simulink model "Architecture"  (R2016b)
settings: Solver=VariableStepAuto  StartTime=0.0  StopTime=10.0  RelTol=1e-3
settings Model: Creator=Taeke  LastModifiedBy=Taeke

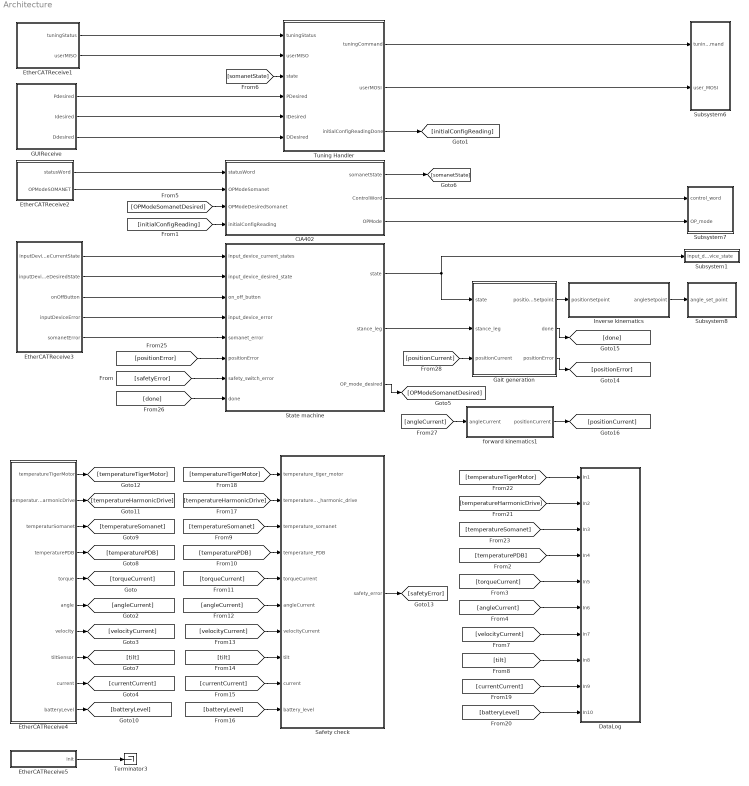
== system Architecture ==
  CiA402 : MATLAB Function  TreatAsAtomicUnit=on
  DataLog : Subsystem
  EtherCATReceive1 : Subsystem
  EtherCATReceive2 : Subsystem
  EtherCATReceive3 : Subsystem
  EtherCATReceive4 : Subsystem
  EtherCATReceive5 : Subsystem
  GUIReceive : Subsystem
  Gait generation : MATLAB Function  TreatAsAtomicUnit=on
  Inverse kinematics : MATLAB Function  TreatAsAtomicUnit=on
  Safety check : MATLAB Function  TreatAsAtomicUnit=on
  State machine : MATLAB Function  TreatAsAtomicUnit=on
  Subsystem1 : Subsystem
  Subsystem6 : Subsystem
  Subsystem7 : Subsystem
  Subsystem8 : Subsystem
  Terminator3 : Terminator
  Tuning Handler : MATLAB Function  TreatAsAtomicUnit=on
  forward kinematics1 : MATLAB Function  TreatAsAtomicUnit=on
  wires:
  EtherCATReceive4/6(angle) -> [angleCurrent]
  EtherCATReceive4/7(velocity) -> [velocityCurrent]
  EtherCATReceive4/8(tiltSensor) -> [tilt]
  EtherCATReceive4/9(current) -> [currentCurrent]
  EtherCATReceive3/3(onOffButton) -> State machine/3(on_off_button)
  EtherCATReceive3/5(somanetError) -> State machine/5(somanet_error)
  EtherCATReceive3/1(inputDeviceCurrentState) -> State machine/1(input_device_current_states)
  EtherCATReceive3/2(inputDeviceDesiredState) -> State machine/2(input_device_desired_state)
  EtherCATReceive3/4(inputDeviceError) -> State machine/4(input_device_error)
  State machine/1(state) -> Gait generation/1(state), Subsystem1/1(input_device_state)
  State machine/2(stance_leg) -> Gait generation/2(stance_leg)
  Gait generation/1(positionSetpoint) -> Inverse kinematics/1(positionSetpoint)
  Inverse kinematics/1(angleSetpoint) -> Subsystem8/1(angle_set_point)
  CiA402/2(ControlWord) -> Subsystem7/1(control_word)
  CiA402/3(OPMode) -> Subsystem7/2(OP_mode)
  EtherCATReceive1/2(userMISO) -> Tuning Handler/2(userMISO)
  EtherCATReceive2/1(statusWord) -> CiA402/1(statusWord)
  EtherCATReceive2/2(OPModeSOMANET) -> CiA402/2(OPModeSomanet)
  [OPModeSomanetDesired] -> CiA402/3(OPModeDesiredSomanet)
  State machine/3(OP_mode_desired) -> [OPModeSomanetDesired]
  CiA402/1(somanetState) -> [somanetState]
  [somanetState] -> Tuning Handler/3(state)
  EtherCATReceive1/1(tuningStatus) -> Tuning Handler/1(tuningStatus)
  EtherCATReceive5/1(init) -> Terminator3/1
  Tuning Handler/2(userMOSI) -> Subsystem6/2(user_MOSI)
  Tuning Handler/1(tuningCommand) -> Subsystem6/1(tuning_command)
  GUIReceive/1(Pdesired) -> Tuning Handler/4(PDesired)
  GUIReceive/3(Ddesired) -> Tuning Handler/6(DDesired)
  GUIReceive/2(Idesired) -> Tuning Handler/5(IDesired)
  Tuning Handler/3(initialConfigReadingDone) -> [initialConfigReading]
  [initialConfigReading] -> CiA402/4(initialConfigReading)
  EtherCATReceive4/3(temperaturSomanet) -> [temperatureSomanet]
  EtherCATReceive4/4(temperaturePDB) -> [temperaturePDB]
  EtherCATReceive4/5(torque) -> [torqueCurrent]
  [temperatureSomanet] -> Safety check/3(temperature_somanet)
  [temperaturePDB] -> Safety check/4(temperature_PDB)
  [torqueCurrent] -> Safety check/5(torqueCurrent)
  [batteryLevel] -> Safety check/10(battery_level)
  [currentCurrent] -> Safety check/9(current)
  [tilt] -> Safety check/8(tilt)
  [velocityCurrent] -> Safety check/7(velocityCurrent)
  [angleCurrent] -> Safety check/6(angleCurrent)
  EtherCATReceive4/10(batteryLevel) -> [batteryLevel]
  EtherCATReceive4/2("temperatureHarmonicDrive ") -> [temperatureHarmonicDrive]
  [temperatureHarmonicDrive] -> Safety check/2(temperature_harmonic_drive)
  EtherCATReceive4/1(temperatureTigerMotor) -> [temperatureTigerMotor]
  [temperatureTigerMotor] -> Safety check/1(temperature_tiger_motor)
  [temperatureTigerMotor] -> DataLog/1(In1)
  [temperatureHarmonicDrive] -> DataLog/2(In2)
  [temperatureSomanet] -> DataLog/3(In3)
  [temperaturePDB] -> DataLog/4(In4)
  [torqueCurrent] -> DataLog/5(In5)
  [angleCurrent] -> DataLog/6(In6)
  [velocityCurrent] -> DataLog/7(In7)
  [tilt] -> DataLog/8(In8)
  [currentCurrent] -> DataLog/9(In9)
  [batteryLevel] -> DataLog/10(In10)
  [positionError] -> State machine/6(positionError)
  Safety check/1(safety_error) -> [safetyError]
  [safetyError] -> State machine/7(safety_switch_error)
  Gait generation/2(done) -> [done]
  Gait generation/3(positionError) -> [positionError]
  [done] -> State machine/8(done)
  [angleCurrent] -> forward kinematics1/1(angleCurrent)
  forward kinematics1/1(positionCurrent) -> [positionCurrent]
  [positionCurrent] -> Gait generation/3(positionCurrent)

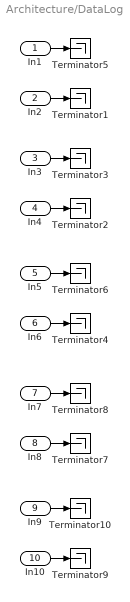
== system Architecture/DataLog ==
  In1 : Inport
  In2 : Inport  Port=2
  In3 : Inport  Port=3
  In4 : Inport  Port=4
  In5 : Inport  Port=5
  In6 : Inport  Port=6
  In7 : Inport  Port=7
  In8 : Inport  Port=8
  In9 : Inport  Port=9
  In10 : Inport  Port=10
  Terminator{1..10} (10 alike) : Terminator
  wires:
  In1/1 -> Terminator5/1
  In2/1 -> Terminator1/1
  In3/1 -> Terminator3/1
  In4/1 -> Terminator2/1
  In5/1 -> Terminator6/1
  In6/1 -> Terminator4/1
  In7/1 -> Terminator8/1
  In8/1 -> Terminator7/1
  In9/1 -> Terminator10/1
  In10/1 -> Terminator9/1

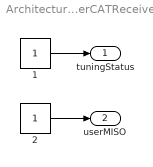
== system Architecture/EtherCATReceive1 ==
  1 : Constant
  2 : Constant
  tuningStatus : Outport
  userMISO : Outport  Port=2
  wires:
  2/1 -> userMISO/1
  1/1 -> tuningStatus/1

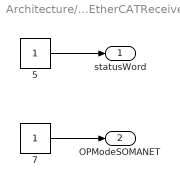
== system Architecture/EtherCATReceive2 ==
  5 : Constant
  7 : Constant
  statusWord : Outport
  OPModeSOMANET : Outport  Port=2
  wires:
  7/1 -> OPModeSOMANET/1
  5/1 -> statusWord/1

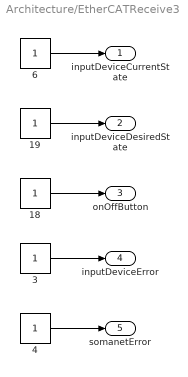
== system Architecture/EtherCATReceive3 ==
  {3..4,6,18..19} (5 alike) : Constant
  inputDeviceCurrentState : Outport
  inputDeviceDesiredState : Outport  Port=2
  onOffButton : Outport  Port=3
  inputDeviceError : Outport  Port=4
  somanetError : Outport  Port=5
  wires:
  18/1 -> onOffButton/1
  19/1 -> inputDeviceDesiredState/1
  3/1 -> inputDeviceError/1
  4/1 -> somanetError/1
  6/1 -> inputDeviceCurrentState/1

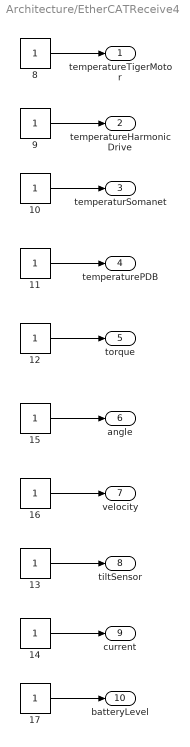
== system Architecture/EtherCATReceive4 ==
  {8..17} (10 alike) : Constant
  temperatureTigerMotor : Outport
  "temperatureHarmonicDrive " : Outport  Port=2
  temperaturSomanet : Outport  Port=3
  temperaturePDB : Outport  Port=4
  torque : Outport  Port=5
  angle : Outport  Port=6
  velocity : Outport  Port=7
  tiltSensor : Outport  Port=8
  current : Outport  Port=9
  batteryLevel : Outport  Port=10
  wires:
  10/1 -> temperaturSomanet/1
  12/1 -> torque/1
  8/1 -> temperatureTigerMotor/1
  11/1 -> temperaturePDB/1
  9/1 -> "temperatureHarmonicDrive "/1
  13/1 -> tiltSensor/1
  17/1 -> batteryLevel/1
  14/1 -> current/1
  16/1 -> velocity/1
  15/1 -> angle/1

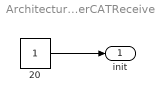
== system Architecture/EtherCATReceive5 ==
  20 : Constant
  init : Outport
  wires:
  20/1 -> init/1

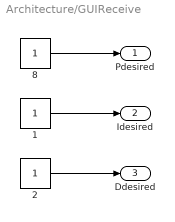
== system Architecture/GUIReceive ==
  1 : Constant
  2 : Constant
  8 : Constant
  Pdesired : Outport
  Idesired : Outport  Port=2
  Ddesired : Outport  Port=3
  wires:
  8/1 -> Pdesired/1
  1/1 -> Idesired/1
  2/1 -> Ddesired/1

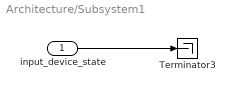
== system Architecture/Subsystem1 ==
  input_device_state : Inport
  Terminator3 : Terminator
  wires:
  input_device_state/1 -> Terminator3/1

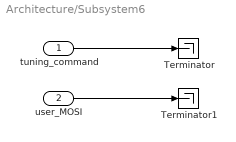
== system Architecture/Subsystem6 ==
  tuning_command : Inport
  user_MOSI : Inport  Port=2
  Terminator : Terminator
  Terminator1 : Terminator
  wires:
  tuning_command/1 -> Terminator/1
  user_MOSI/1 -> Terminator1/1

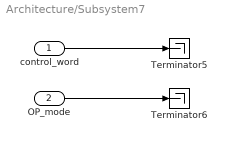
== system Architecture/Subsystem7 ==
  control_word : Inport
  OP_mode : Inport  Port=2
  Terminator5 : Terminator
  Terminator6 : Terminator
  wires:
  control_word/1 -> Terminator5/1
  OP_mode/1 -> Terminator6/1

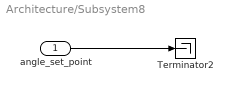
== system Architecture/Subsystem8 ==
  angle_set_point : Inport
  Terminator2 : Terminator
  wires:
  angle_set_point/1 -> Terminator2/1

== matlab function Architecture/State machine ==
  data: state output; stance_leg output; OP_mode_desired output; input_device_current_states input; input_device_desired_state input; on_off_button input; input_device_error input; somanet_error input; positionError input; safety_switch_error input; done input
function [state, stance_leg, OP_mode_desired] = state_machine(input_device_current_states, input_device_desired_state,  on_off_button,input_device_error, somanet_error, positionError, safety_switch_error, done)

y = u;
end

== matlab function Architecture/Tuning Handler ==
  data: tuningStatus input; tuningCommand output; userMISO input; userMOSI output; state input; PDesired input; IDesired input; DDesired input; initialConfigReadingDone output
function [tuningCommand, userMOSI, initialConfigReadingDone] = tuning_handler(tuningStatus, userMISO, state, PDesired, IDesired, DDesired)

end

== matlab function Architecture/Safety check ==
  data: temperature_tiger_motor input; safety_error output; temperature_harmonic_drive input; temperature_somanet input; temperature_PDB input; torqueCurrent input; angleCurrent input; velocityCurrent input; tilt input; current input; battery_level input
function safety_error  = safety_check(temperature_tiger_motor, temperature_harmonic_drive, temperature_somanet, temperature_PDB, torqueCurrent, angleCurrent, velocityCurrent, tilt, current, battery_level)

end

== matlab function Architecture/CiA402 ==
  data: somanetState output; statusWord input; ControlWord output; OPModeSomanet input; OPModeDesiredSomanet input; OPMode output; initialConfigReading input
function [somanetState, ControlWord, OPMode] = CiA402(statusWord, OPModeSomanet, OPModeDesiredSomanet, initialConfigReading)
end

== matlab function Architecture/Gait generation ==
  data: positionSetpoint output; state input; stance_leg input; done output; positionCurrent input; positionError output
function [positionSetpoint,done, positionError] = gait_generation(state, stance_leg, positionCurrent)

y = u;
end

== matlab function Architecture/Inverse kinematics ==
  data: positionSetpoint input; angleSetpoint output
function angleSetpoint  = inverse_kinematics(positionSetpoint)

end

== matlab function Architecture/forward kinematics1 ==
  data: angleCurrent input; positionCurrent output
function positionCurrent  = forward_kinematics(angleCurrent)

end
